simulink model "FIR_LMS_2"  (R2019b)
settings: Solver=VariableStepDiscrete  StartTime=0.0  StopTime=100e-6  RelTol=1e-3
libraries: xbsIndex_r4 x55
settings Model: Creator=blaisvin  LastModifiedBy=blaisvin

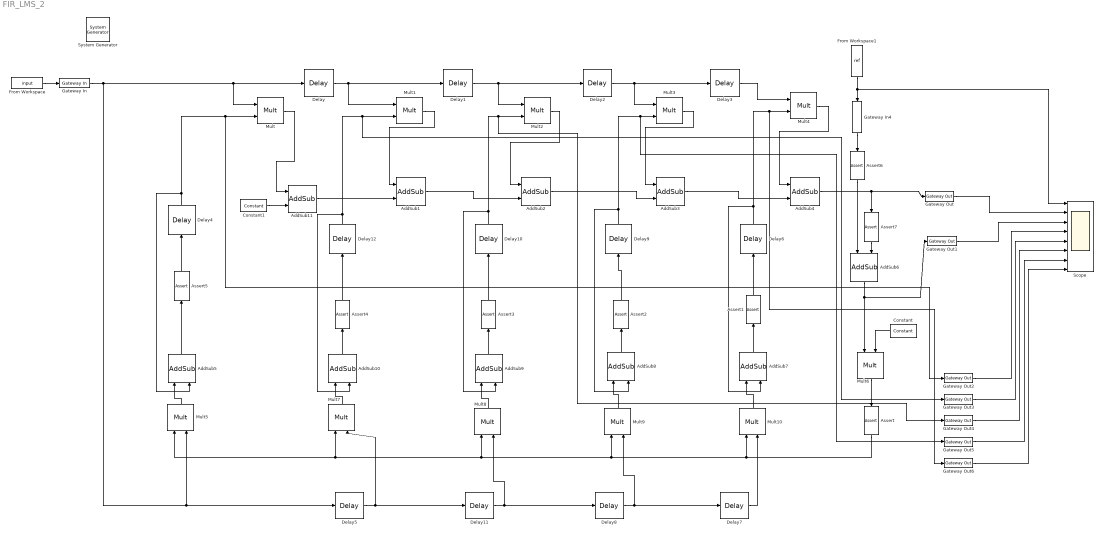
== system FIR_LMS_2 ==
  " System Generator" : xbsIndex_r4/ System Generator  Tag=genX  xilinxfamily=kintex7  part=xc7k325t  speed=-3  package=fbg676  synthesis_tool=Vivado  clock_wrapper=Clock Enables  directory=./netlist  proj_type=Vivado  Synth_file=Vivado Synthesis Defaults  Impl_file=Vivado Implementation Defaults  testbench=on  simulink_period=1/20e6  sysclk_period=50  dcm_input_clock_period=10  incr_netlist=off  trim_vbits=Everywhere in SubSystem  dbl_ovrd=According to Block Masks  core_generation=According to Block Masks  run_coregen=off  deprecated_control=off  eval_field=0  block_type=sysgen
  AddSub{1..3,11} (4 alike) : xbsIndex_r4/AddSub  mode=Addition  use_carryin=off  use_carryout=off  en=off  latency=0  precision=User Defined  arith_type=Unsigned  n_bits=16  bin_pt=14  quantization=Truncate  overflow=Wrap  use_behavioral_HDL=off  hw_selection=Fabric  pipelined=off  dbl_ovrd=off  block_type=addsub
  AddSub{4..5,7..10} (6 alike) : xbsIndex_r4/AddSub  mode=Addition  use_carryin=off  use_carryout=off  en=off  latency=0  precision=User Defined  arith_type="Signed  (2's comp)"  n_bits=16  bin_pt=14  quantization=Truncate  overflow=Wrap  use_behavioral_HDL=off  hw_selection=Fabric  pipelined=off  dbl_ovrd=off  block_type=addsub
  AddSub6 : xbsIndex_r4/AddSub  mode=Subtraction  use_carryin=off  use_carryout=off  en=off  latency=0  precision=User Defined  arith_type="Signed  (2's comp)"  n_bits=16  bin_pt=14  quantization=Truncate  overflow=Wrap  use_behavioral_HDL=off  hw_selection=Fabric  pipelined=off  dbl_ovrd=off  block_type=addsub
  Assert{,1..7} (8 alike) : xbsIndex_r4/Assert  assert_type=on  type_source=Explicitly  gui_display_data_type=Fixed-point  arith_type="Signed  (2's comp)"  n_bits=16  bin_pt=14  preci_type=Single  exp_width=8  frac_width=24  assert_rate=on  rate_source=Explicitly  period=1/20e6  output_port=on  block_type=assert
  Constant : xbsIndex_r4/Constant  const=0.25  gui_display_data_type=Fixed-point  arith_type=Signed (2's comp)  n_bits=16  bin_pt=14  preci_type=Single  exp_width=8  frac_width=24  explicit_period=off  period=1  equ=P=C  opselect=C  inp2=PCIN>>17  opr=+  inp1=P  carry=CIN  dbl_ovrd=off  block_type=constant
  Constant1 : xbsIndex_r4/Constant  const=0  gui_display_data_type=Fixed-point  arith_type=Signed (2's comp)  n_bits=16  bin_pt=14  preci_type=Single  exp_width=8  frac_width=24  explicit_period=off  period=1  equ=P=C  opselect=C  inp2=PCIN>>17  opr=+  inp1=P  carry=CIN  dbl_ovrd=off  block_type=constant
  Delay{,1..12} (13 alike) : xbsIndex_r4/Delay  rst=off  infoeditControl=Selection of Reset will increase slice count due to use of real FFs and instead of SRLs  en=off  latency=1  reg_retiming=off  dbl_ovrd=off  block_type=delay
  From Workspace : FromWorkspace  VariableName=input  SampleTime=0
  From Workspace1 : FromWorkspace  VariableName=ref  SampleTime=0
  Gateway In : xbsIndex_r4/Gateway In  gui_display_data_type=Fixed-point  arith_type="Signed  (2's comp)"  n_bits=16  bin_pt=14  preci_type=Single  exp_width=8  frac_width=24  rows=1  columns=1  quantization="Round  (unbiased: +/- Inf)"  overflow=Saturate  period=1/20e6  UseAsADC=off  ADCChannel='1'  interface=None  automatic_assignment=on  address_offset=hex2dec('00')  intf_name=''  intf_description=''  default_value=0  timing_constraint=None  locs_specified=off  LOCs={}  io_standard={}  inherit_from_input=off  hdl_port=on  dbl_ovrd=off  block_type=gatewayin
  Gateway In4 : xbsIndex_r4/Gateway In  gui_display_data_type=Fixed-point  arith_type="Signed  (2's comp)"  n_bits=16  bin_pt=14  preci_type=Single  exp_width=8  frac_width=24  rows=1  columns=1  quantization="Round  (unbiased: +/- Inf)"  overflow=Saturate  period=1/20e6  UseAsADC=off  ADCChannel='1'  interface=None  automatic_assignment=on  address_offset=hex2dec('00')  intf_name=''  intf_description=''  default_value=0  timing_constraint=None  locs_specified=off  LOCs={}  io_standard={}  inherit_from_input=off  hdl_port=on  dbl_ovrd=off  block_type=gatewayin
  Gateway Out{,1..6} (7 alike) : xbsIndex_r4/Gateway Out  inherit_from_input=off  hdl_port=on  rows=1  columns=1  UseAsDAC=off  DACChannel='1'  interface=None  automatic_assignment=on  address_offset=hex2dec('00')  intf_name=''  intf_description=''  timing_constraint=None  locs_specified=off  LOCs={}  io_standard={}  block_type=gatewayout
  Mult{,1..10} (11 alike) : xbsIndex_r4/Mult  precision=User Defined  arith_type="Signed  (2's comp)"  n_bits=16  bin_pt=14  quantization=Truncate  overflow=Wrap  en=off  latency=0  use_behavioral_HDL=off  opt=Speed  use_embedded=on  optimum_pipeline=off  pipeline=on  dbl_ovrd=off  use_rpm=on  placement_style=Triangular  block_type=mult
  Scope : Scope  NumInputPorts=8
  wires:
  AddSub1/1 -> AddSub2/2
  Gateway In/1 -> Mult5/2, Delay5/1, Mult/1, Delay/1
  AddSub2/1 -> AddSub3/2
  Mult4/1 -> AddSub4/1
  From Workspace/1 -> Gateway In/1
  Mult1/1 -> AddSub1/1
  Delay2/1 -> Delay3/1, Mult3/1
  Delay1/1 -> Mult2/1, Delay2/1
  Mult2/1 -> AddSub2/1
  Delay3/1 -> Mult4/1
  AddSub3/1 -> AddSub4/2
  Mult3/1 -> AddSub3/1
  Delay/1 -> Mult1/1, Delay1/1
  AddSub5/1 -> Assert5/1
  Mult5/1 -> AddSub5/1
  AddSub4/1 -> Assert7/1, Gateway Out/1
  From Workspace1/1 -> Gateway In4/1, Scope/1
  Constant/1 -> Mult6/2
  Mult10/1 -> AddSub7/1
  Mult6/1 -> Assert/1
  Delay7/1 -> Mult10/2
  Delay8/1 -> Delay7/1, Mult9/2
  Mult9/1 -> AddSub8/1
  Mult8/1 -> AddSub9/1
  Delay11/1 -> Delay8/1, Mult8/2
  Delay5/1 -> Delay11/1, Mult7/2
  Mult7/1 -> AddSub10/1
  Gateway Out/1 -> Scope/2
  Delay4/1 -> Gateway Out2/1, Mult/2, AddSub5/2
  Delay12/1 -> Gateway Out3/1, Mult1/2, AddSub10/2
  Delay10/1 -> Gateway Out4/1, Mult2/2, AddSub9/2
  Delay9/1 -> Gateway Out5/1, Mult3/2, AddSub8/2
  Delay6/1 -> Gateway Out6/1, Mult4/2, AddSub7/2
  AddSub11/1 -> AddSub1/2
  Mult/1 -> AddSub11/1
  Constant1/1 -> AddSub11/2
  AddSub6/1 -> Gateway Out1/1, Mult6/1
  Gateway Out1/1 -> Scope/3
  Gateway Out2/1 -> Scope/4
  Gateway Out3/1 -> Scope/5
  Gateway Out4/1 -> Scope/6
  Gateway Out5/1 -> Scope/7
  Gateway Out6/1 -> Scope/8
  Assert/1 -> Mult5/1, Mult7/1, Mult8/1, Mult9/1, Mult10/1
  Assert5/1 -> Delay4/1
  AddSub10/1 -> Assert4/1
  Assert4/1 -> Delay12/1
  Assert3/1 -> Delay10/1
  AddSub9/1 -> Assert3/1
  AddSub8/1 -> Assert2/1
  Assert2/1 -> Delay9/1
  AddSub7/1 -> Assert1/1
  Assert1/1 -> Delay6/1
  Gateway In4/1 -> Assert6/1
  Assert6/1 -> AddSub6/1
  Assert7/1 -> AddSub6/2
